simulink model "SimpleODEwithInp"  (R2016a)
settings: Solver=ode45  StartTime=0.0  StopTime=10.0  MaxStep=0.1  RelTol=1e-3
settings Model: Creator=gfaineko  LastModifiedBy=georgios
settings DataIOCC: SaveFormat=Array  DSMLogging=off
settings DebuggingCC: UnderspecifiedInitializationDetection=Classic  MergeDetectMultiDrivingBlocksExec=none  SolverPrmCheckMsg=warning  StateNameClashWarn=warning
settings HardwareCC: ProdBitPerPointer=32  ProdLargestAtomicFloat=None  ProdIntDivRoundTo=Undefined  ProdEndianess=Unspecified  ProdWordSize=32  ProdHWDeviceType=32-bit Generic
settings ModelReferenceCC: PropagateSignalLabelsOutOfModel=off
settings ConfigComp: CovModelRefEnable=Off

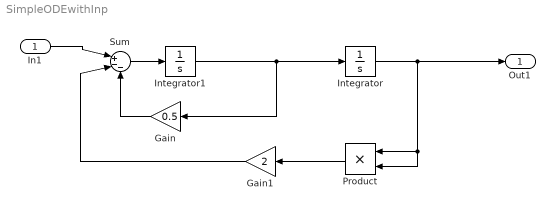
== system SimpleODEwithInp ==
  In1 : Inport
  Gain : Gain  Gain=0.5
  Gain1 : Gain  Gain=2
  Integrator : Integrator
  Integrator1 : Integrator
  Product : Product
  Sum : Sum  Inputs=|+--
  Out1 : Outport
  wires:
  Integrator/1 -> Product/2, Product/1, Out1/1
  In1/1 -> Sum/1
  Sum/1 -> Integrator1/1
  Gain1/1 -> Sum/2
  Gain/1 -> Sum/3
  Integrator1/1 -> Gain/1, Integrator/1
  Product/1 -> Gain1/1
